simulink model "Prob3"  (R2020b)
settings: Solver=VariableStepAuto  StartTime=0.0  StopTime=10.0  RelTol=1e-3
settings Model: Creator=shoun  LastModifiedBy=shoun

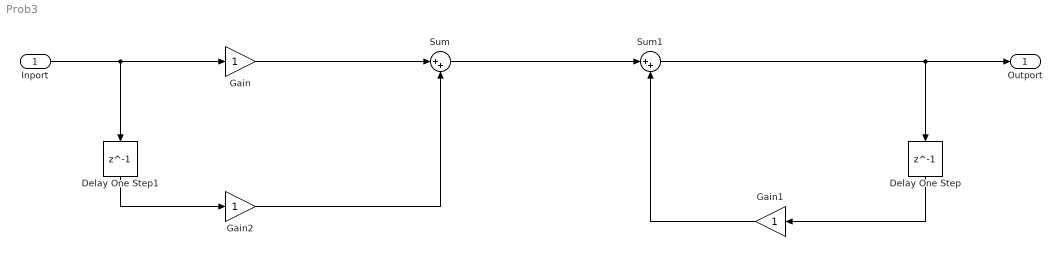
== system Prob3 ==
  Inport : Inport
  Delay One Step : Delay  DelayLength=1
  Delay One Step1 : Delay  DelayLength=1
  Gain : Gain
  Gain1 : Gain
  Gain2 : Gain
  Sum : Sum  Inputs=|++
  Sum1 : Sum  Inputs=|++
  Outport : Outport
  wires:
  Sum1/1 -> Delay One Step/1, Outport/1
  Delay One Step/1 -> Gain1/1
  Gain1/1 -> Sum1/2
  Sum/1 -> Sum1/1
  Inport/1 -> Delay One Step1/1, Gain/1
  Gain/1 -> Sum/1
  Delay One Step1/1 -> Gain2/1
  Gain2/1 -> Sum/2
